simulink model "CRANE2D"  (R2018a)
settings: Solver=VariableStepAuto  StartTime=0.0  StopTime=500.0  RelTol=1e-3
undefined symbols (not defined in the file or in its folder): sigbuilder_block
settings Model: Creator=mural  LastModifiedBy=mural

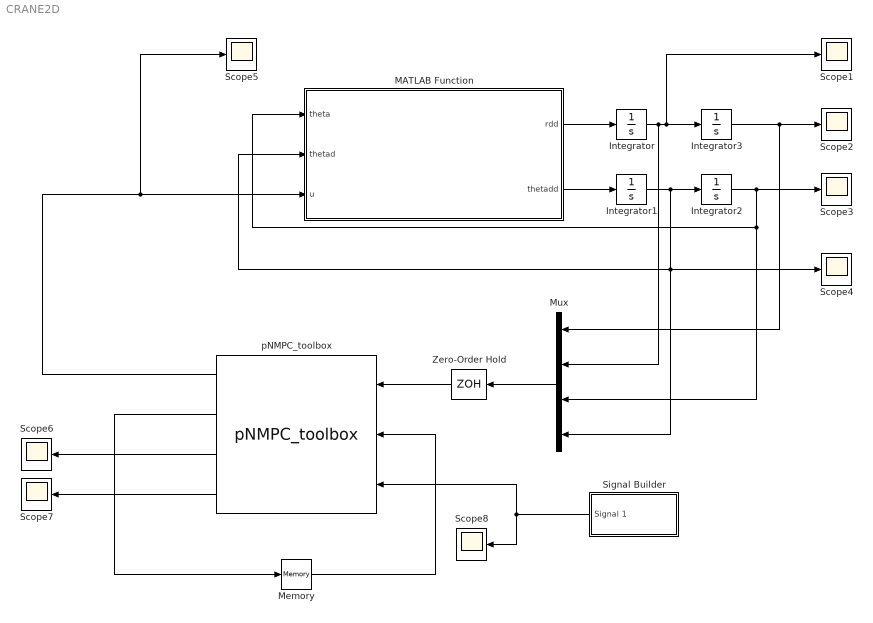
== system CRANE2D ==
  Integrator{,1..3} (4 alike) : Integrator
  MATLAB Function : MATLAB Function  TreatAsAtomicUnit=on
  Memory : Memory
  Mux : Mux
  Scope{1..8} (8 alike) : Scope
  Signal Builder : Subsystem  Tag=STV Subsys  LoadFcn=sigbuilder_block('load');  StartFcn=sigbuilder_block('start');  StopFcn=sigbuilder_block('stop');  ClipboardFcn=sigbuilder_block('clipboard');  mask(Sigbuilder block){tuvar=[0:10]}
      mask help: Simulink:masks:SigbuilderBlock_MD
      mask init:
      | if ~strcmp(get_param(bdroot(gcbh),'SimulationStatus'),'stopped') tuvar = sigbuilder_block('maskInit'); end
      settings: CopyFcn=sigbuilder_block('copy');  DeleteFcn=sigbuilder_block('delete');  ModelCloseFcn=sigbuilder_block('modelClose');  PreSaveFcn=sigbuilder_block('preSave');  PauseFcn=sigbuilder_block('pause');  ContinueFcn=sigbuilder_block('continue');  NameChangeFcn=sigbuilder_block('namechange');  OpenFcn=sigbuilder_block('open',[-1339.8 -80.4 1141.2 522.6 ]);  CloseFcn=sigbuilder_block('close');
      mask Display: plot(0, 0, 100, 100,[2, 2, 32, 32, 2], [68, 8, 8, 68, 68],[32, 2], [38, 38], [32, 19, 2],[53, 60, 44], [32, 17, 17, 2],[16, 16, 31, 31]);txt = getActiveGroup(gcbh);text(2, 100, txt,'verticalAlignment', 'top');
  Zero-Order Hold : ZeroOrderHold  SampleTime=0.1
  pNMPC_toolbox : S-Function  FunctionName=pNMPC_toolbox  SFunctionDeploymentMode=off  EnableBusSupport=off  mask(Legacy Function){SFunctionSpec=BBO_SQP(Real_C u1[4],Real_C u2[5],Real_C u3[1],Real_C y1[1],Real_C y2[5],Real_C y3[1],Real_C y4[1]), ShowSpec=on}
      mask prompts: ShowSpec "Display function specification"
      mask help:
      | This block allows you to call the legacy functions specified by the following Legacy Code Tool definition:
      | def.SFunctionName = 'pNMPC_toolbox';
      | def.OutputFcnSpec = 'BBO_SQP(Real_C u1[4],Real_C u2[5],Real_C u3[1],Real_C y1[1],Real_C y2[5],Real_C y3[1],Real_C y4[1])';
      | def.HeaderFiles = {'SQPInterfaceSFUN.h', 'BBOSQPCONSTCall.h', 'BBOSQPOBJCall.h', 'RegularConstraints.h', 'TerminalConstraints.h', 'Dynamics.h', 'Lagrangian.h', 'Mayer.h', 'PNMPC_SQP.h', 'SQP_BBO.h', 'ParameterInputMap.h', 'PNMPC_ROOT.h', 'ControlClockLinear.h', 'ControlClockPiecewise.h', 'Integrator_RK45.h', 'Integrator_EU.h', 'Integrator_HEUN.h'};
      | def.SourceFiles = {'SQPInterfaceSFUN.c', 'BBOSQPCONSTCall.c', 'BBOSQPOBJCall.c', 'RegularConstraints.c', 'TerminalConstraints.c', 'Dynamics.c', 'Lagrangian.c', 'Mayer.c', 'PNMPC_SQP.c', 'SQP_BBO.c', 'ParameterInputMap.c'};
      | def.IncPaths = {'F:\LoEMarch\MATLAB_STREAM\CCODEGEN\include', 'F:\LoEMarch\MATLAB_STREAM\pNMPC\Integrators', 'F:\LoEMarch\MATLAB_STREAM\pNMPC\Parameterization', 'F:\LoEMarch\MATLAB_STREAM\pNMPC\Solver'};
      mask init:
      | set_param('CRANE2D/pNMPC_toolbox', 'MaskDisplay', 'disp(''{\bf\fontsize{40}\fontname{Microsoft Himalaya}pNMPC}'', ''texmode'',''on''), port_label(''input'',1,''X0[4]'');port_label(''input'',2,''U_PARAM_W[5]'');port_label(''input'',3,''P[1]'');port_label(''output'',1,''U_ACT[1]'');port_label(''output'',2,''U_PARAM[5]'');port_label(''output'',3,''CompTime'');port_label(''output'',4,''OBJ'');')
      mask Help: <p>This block was generated automatically by the Legacy Code Tool. For detailed help on this tool, call<a href="matlab:legacy_code('help')"> legacy_code('help')</a>.</p>
      mask Callback ShowSpec:
      | if strcmp(get_param(gcbh, 'ShowSpec'), 'on')
      |   set_param(gcbh, 'MaskDisplay', sprintf('fprintf(''%s'');', get_param(gcbh, 'SFunctionSpec')));
      | else
      |   set_param(gcbh, 'MaskDisplay', sprintf('fprintf(''%s'');', get_param(gcbh, 'FunctionName')));
      | end
      mask Display: disp('{\bf\fontsize{40}\fontname{Microsoft Himalaya}pNMPC}', 'texmode','on'), port_label('input',1,'X0[4]');port_label('input',2,'U_PARAM_W[5]');port_label('input',3,'P[1]');port_label('output',1,'U_ACT[1]');port_label('output',2,'U_PARAM[5]');port_label('output',3,'CompTime');port_label('output',4,'OBJ');
  wires:
  Mux/1 -> Zero-Order Hold/1
  MATLAB Function/1(rdd) -> Integrator/1
  MATLAB Function/2(thetadd) -> Integrator1/1
  Integrator1/1 -> Mux/4, MATLAB Function/2(thetad), Scope4/1, Integrator2/1
  Integrator/1 -> Integrator3/1, Scope1/1, Mux/2
  Integrator3/1 -> Mux/1, Scope2/1
  Integrator2/1 -> MATLAB Function/1(theta), Mux/3, Scope3/1
  Zero-Order Hold/1 -> pNMPC_toolbox/1
  Memory/1 -> pNMPC_toolbox/2
  pNMPC_toolbox/3 -> Scope6/1
  pNMPC_toolbox/4 -> Scope7/1
  Signal Builder/1(Signal 1) -> pNMPC_toolbox/3, Scope8/1
  pNMPC_toolbox/1 -> Scope5/1, MATLAB Function/3(u)
  pNMPC_toolbox/2 -> Memory/1

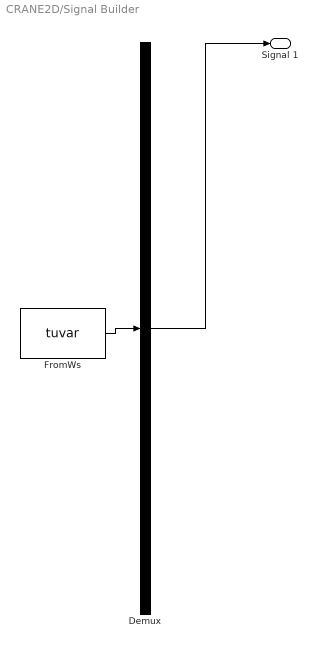
== system CRANE2D/Signal Builder ==
  Demux : Demux  Tag=STV Demux  Outputs=1
  FromWs : FromWorkspace  Tag=STV FromWs  VariableName=tuvar  SampleTime=0
      SigBuilderData=|
      | common.afterFinalStr = 'Extrapolate'
      | common.sampleTime = 0
      | dataSet.timeRange = [0 200]
      | dataSet.name = 'Group 1'
      | sbobj.Groups.Name = 'Group 1'
      | sbobj.Groups.Signals.Name = 'Signal 1'
      | sbobj.Groups.Signals.XData = [0 53 53 93.6 93.6 140 140 180.2 180.2 200]
      | sbobj.Groups.Signals.YData = [4 4 0 0 -4 -4 0 0 2.98 2.98]
      | sbobj.Groups.TimeRange = [0 200]
  Signal 1 : Outport  Tag=STV Outport
  wires:
  Demux/1 -> Signal 1/1
  FromWs/1 -> Demux/1

== matlab function CRANE2D/MATLAB Function ==
  data: theta input; rdd output; thetad input; u input; thetadd output
function [rdd,thetadd] = fcn(theta,thetad,u)
% Parameters
 m = 200; M = 1500; l = 100; fr = 10^5; g = 9.81; 
 % Dynamics 
rdd = (u + m*g*cos(theta)*sin(theta) + m*l*thetad*thetad*sin(theta))/(M + m*(1-(cos(theta)*cos(theta))));
thetadd = (-u*cos(theta) - m*l*thetad*thetad*cos(theta)*sin(theta) - (M-m)*g*sin(theta) - fr*thetad)/((M + m*sin(theta)*sin(theta))*l);
